simulink model "SmAHTR_r1_PITTRTNUKE"  (R2014a)
settings: Solver=ode4  StartTime=0.0  StopTime=250  FixedStep=.001  RelTol=1e-3
PreLoadFcn:
  | load DarkLowerCoeffs
  | load DarkMiddleCoeffs
  | load DarkUpperCoeffs
  | load breaks
values from neighbouring files (symbols this model uses):
  alpha = [ -2.61*pcm -0.53*pcm ]    [SmAHTR_Spatial_Kinetics.m]
  breaks = DarkLowerBreaks    [SmAHTR_Spatial_Kinetics.m]
  cpc = 2414    [SmAHTR_Spatial_Kinetics.m]
  cpp = 2414    [SmAHTR_Spatial_Kinetics.m]
  DarkLowerCoeffs = ppDarkLower.coefs    [SmAHTR_Spatial_Kinetics.m]
  DarkMiddleCoeffs = ppDarkMiddle.coefs    [SmAHTR_Spatial_Kinetics.m]
  DarkRodWorthInserted = -3*Beta    (= -0.00489)    [SmAHTR_Spatial_Kinetics.m]
  DarkUpperCoeffs = ppDarkUpper.coefs    [SmAHTR_Spatial_Kinetics.m]
  delta_t = 1 / sensor_sampling_rate    (= 0.001)    [HeatExchanger_ps.m]    (also in steady_data_76rssi_30_1.mat = 0.1; steady_data_76rssi_40.mat = 0.1; steady_data_76rssi_iter.mat = 0.1; steady_data_76rssi_iter_reduce.mat = 0.1)
  Kc1 = 1/(rho_secondary*V_secondary)    (= 0.00032726218348)    [SmAHTR_Spatial_Kinetics.m]
  Kc2 = (h_secondary*A)/(cps*rho_secondary*V_secondary)    (= 1.23242359038)    [SmAHTR_Spatial_Kinetics.m]
  Kh1 = 1/(rho_primary*V_primary)    (= 0.000447917898441)    [SmAHTR_Spatial_Kinetics.m]
  Kh2 = (h_primary*A)/(cpp*rho_primary*V_primary)    (= 1.29038206968)    [SmAHTR_Spatial_Kinetics.m]
  Kw1 = h_primary    (= 23800)    [SmAHTR_Spatial_Kinetics.m]
  Kw2 = h_secondary    (= 24500)    [SmAHTR_Spatial_Kinetics.m]
  Kw3 = A/(rho_tube*cpw*V_tube)    (= 0.000122049789882)    [SmAHTR_Spatial_Kinetics.m]
  L1 = .0124    (= 0.0124)    [SmAHTR_Spatial_Kinetics.m]
  L2 = .0305    (= 0.0305)    [SmAHTR_Spatial_Kinetics.m]
  rcp_activatetime = 20    [SmAHTR_Spatial_Kinetics.m]
  rcpt = 0.1    [SmAHTR_Spatial_Kinetics.m]
  SaltVaultICs = -AtempSALT\btempSALT*u0    [SmAHTR_Spatial_Kinetics.m]
  Tp_i = 700    [SmAHTR_Spatial_Kinetics.m]
  Ts_i = 600    [SmAHTR_Spatial_Kinetics.m]
  Tw_i = 650    [SmAHTR_Spatial_Kinetics.m]
  xfc0 = -Atemp\btemp*u0    [SmAHTR_Spatial_Kinetics.m]
libraries: powerlib_meascontrol x9, simulink x3
(part 1 of 2)
settings Model: BufferReuse=off  Creator=LabUser  LastModifiedBy=wangwenchen
settings DataIOCC: SignalLoggingSaveFormat=ModelDataLogs
settings OptimizationCC: BlockReduction=off  OptimizeBlockIOStorage=off  BufferReuse=off  GlobalBufferReuse=off  ExpressionFolding=off  LocalBlockOutputs=off
settings DebuggingCC: UnderspecifiedInitializationDetection=Classic  MultiTaskDSMMsg=warning  MultiTaskCondExecSysMsg=none  StateNameClashWarn=warning
settings HardwareCC: ProdIntDivRoundTo=Zero  ProdEndianess=LittleEndian  ProdHWDeviceType=Generic->32-bit x86 compatible
settings RTWCC: ProcessScript=grt_make_rtw_hook  IncludeERTFirstTime=on  RTWCompilerOptimization=On

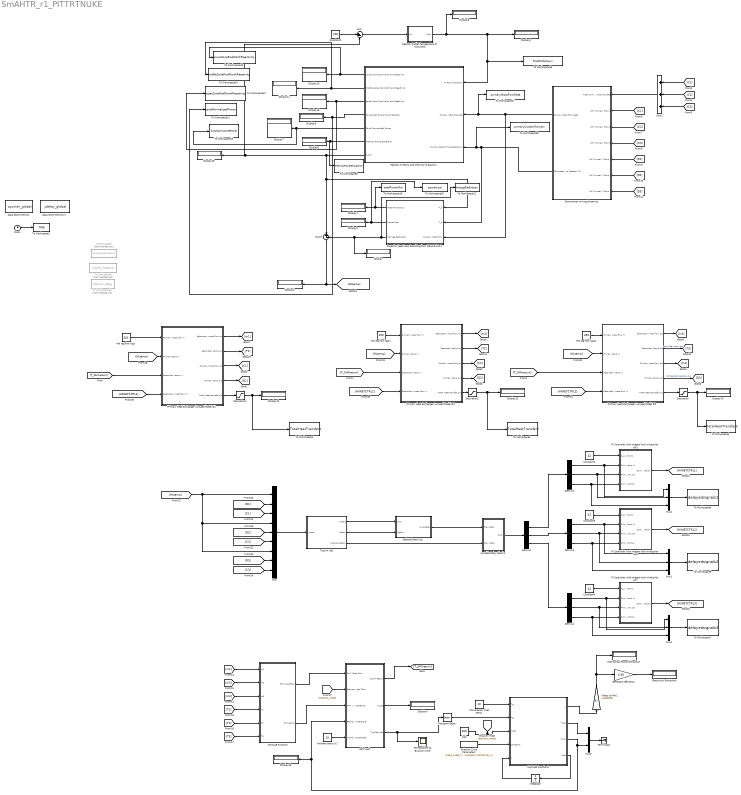
== system SmAHTR_r1_PITTRTNUKE ==
  Ambient temp (C) : Constant  Value=25
  Brayton Cycle Parameters : FromWorkspace  VariableName=[0,eta_C,eta_T,r,cpCO2Turbine,cpCO2Compressor,rhoCO2,tau_t]  SampleTime=0
  Clock : Clock
  Compressor Inlet Temp : Constant  Value=10
  Constant1 : Constant  Value=700
  Constant2 : Constant  Value=42
  Constant3 : Constant  Value=42
  Constant4 : Constant  Value=42
  Data Store Memory : DataStoreMemory  DataStoreName=counter_global  ReadBeforeWriteMsg=warning  WriteAfterWriteMsg=warning  WriteAfterReadMsg=warning  OutDataTypeStr=int32
  Data Store Memory1 : DataStoreMemory  DataStoreName=ydelay_global  ReadBeforeWriteMsg=warning  WriteAfterWriteMsg=warning  WriteAfterReadMsg=warning  InitialValue=ones(10,1)  OutDataTypeStr=int32
  Delayed Data Up2 : MATLAB Function  TreatAsAtomicUnit=on  SystemSampleTime=0.001
  Demux{1..4} (4 alike) : Demux  Outputs=3
  Display{,1..16,18} (18 alike) : Display
  Downcomer mixing dynamics : Subsystem
  Electricity Extraction : Display
  Generator Efficiency : Gain  Gain=0.60
  Hot leg flow kg/s : Constant  Value=350
  Hot leg flow kg/s1 : Constant  Value=350
  Hot leg flow kg/s2 : Constant  Value=350
  Integrator : Integrator
  MATLAB Function : MATLAB Function  TreatAsAtomicUnit=on
  MATLAB Function1 : MATLAB Function  TreatAsAtomicUnit=on
  Mechanical Power Extraction : Display
  Mux : Mux  Inputs=9
  Mux1 : Mux  Inputs=3
  Mux2 : Mux  Inputs=3
  Mux3 : Mux  Inputs=2
  Mux4 : Mux  Inputs=3
  PI Controller with Integral Anti-windup for HX5 : Subsystem
  PI Controller with Integral Anti-windup for HX6 : Subsystem
  PI Controller with Integral Anti-windup for HX7 : Subsystem
  Parasitic Heat Loss Resulting from DRACS HXs1 : Subsystem
  Primary Heat Exchanger Lumped Model #1 : Subsystem
  Primary Heat Exchanger Lumped Model #2 : Subsystem
  Primary Heat Exchanger Lumped Model #3 : Subsystem
  Reactor Kinetics and Thermal Hydraulics : Subsystem
  Reactor Outlet Temperature PI Controller : Subsystem
  Salt Vault : Subsystem
  Saturation : Saturate  UpperLimit=inf  LowerLimit=0
  Saturation1 : Saturate  UpperLimit=inf  LowerLimit=0
  Saturation2 : Saturate  UpperLimit=inf  LowerLimit=0
  Sum : Sum  Inputs=|+-
  Sum1 : Sum  Inputs=+++
  Sum3 : Sum  Inputs=|+-
  Temperature to Brayton cycle : Scope
      settings: SaveName=ScopeData5
  Terminator : Terminator
  To Workspace : ToWorkspace  Commented=on  VariableName=primarytempout  SaveFormat=Timeseries  SampleTime=-1
  To Workspace1 : ToWorkspace  VariableName=TIME  SampleTime=-1
  To Workspace10 : ToWorkspace  VariableName=ZonalNormalizedPower  SaveFormat=Timeseries  SampleTime=-1
  To Workspace11 : ToWorkspace  VariableName=zonalNormalizedPower  SaveFormat=Timeseries  SampleTime=-1
  To Workspace12 : ToWorkspace  VariableName=upperZoneRodWorthReactivity  SaveFormat=Timeseries  SampleTime=-1
  To Workspace13 : ToWorkspace  Commented=on  VariableName=network_delay  SampleTime=-1
  To Workspace14 : ToWorkspace  VariableName=middleZoneRodWorthReactivity  SaveFormat=Timeseries  SampleTime=-1
  To Workspace15 : ToWorkspace  VariableName=lowerZoneRodWorthReactivity  SaveFormat=Timeseries  SampleTime=-1
  To Workspace16 : ToWorkspace  VariableName=RodWithdrawn  SaveFormat=Timeseries  SampleTime=-1
  To Workspace17 : ToWorkspace  VariableName=primaryMassFlowRate  SaveFormat=Timeseries  SampleTime=-1
  To Workspace18 : ToWorkspace  VariableName=primaryCoolantTempIn  SaveFormat=Timeseries  SampleTime=-1
  To Workspace19 : ToWorkspace  VariableName=totalPowerOut  SaveFormat=Timeseries  SampleTime=-1
  To Workspace2 : ToWorkspace  VariableName=TotalHeatTransfer2  SaveFormat=Timeseries  SampleTime=-1
  To Workspace20 : ToWorkspace  VariableName=powerLost  SaveFormat=Timeseries  SampleTime=-1
  To Workspace21 : ToWorkspace  VariableName=hotLegReduction  SaveFormat=Timeseries  SampleTime=-1
  To Workspace3 : ToWorkspace  VariableName=TotalHeatTransfer1  SaveFormat=Timeseries  SampleTime=-1
  To Workspace4 : ToWorkspace  VariableName=TotalHeatTransfer3  SaveFormat=Timeseries  SampleTime=-1
  To Workspace5 : ToWorkspace  Commented=on  VariableName=Signal_measure  SampleTime=-1
  To Workspace6 : ToWorkspace  VariableName=delayedsignals1  SaveFormat=Timeseries  SampleTime=-1
  To Workspace7 : ToWorkspace  VariableName=delayedsignals3  SaveFormat=Timeseries  SampleTime=-1
  To Workspace8 : ToWorkspace  VariableName=delayedsignals2  SaveFormat=Timeseries  SampleTime=-1
  To Workspace9 : ToWorkspace  VariableName=ThermalPowerExtraction  SaveFormat=Timeseries  SampleTime=-1
  Tossim Up1 : MATLAB Function  TreatAsAtomicUnit=on  SystemSampleTime=0.001
  Transport Delay : TransportDelay  DelayTime=0.5  BufferSize=3072
  Variable Delay Block1 : Subsystem
  Watts to MW1 : Gain  Gain=1/1000000
  kg/s : Constant  Value=300
  wires:
  Reactor Outlet Temperature PI Controller/1(Out1) -> Reactor Kinetics and Thermal Hydraulics/1(% Rod Withdrawn), To Workspace16/1, Display5/1, Display8/1
  Downcomer mixing dynamics/1(Primary Mass Flow Rate) -> Parasitic Heat Loss Resulting from DRACS HXs1/3(Primary Mass Flow), To Workspace17/1, Reactor Kinetics and Thermal Hydraulics/2(Primary Mass Flowrate)
  Parasitic Heat Loss Resulting from DRACS HXs1/3(Hot Leg Reduction) -> Sum3/2, Display/1, To Workspace21/1
  Parasitic Heat Loss Resulting from DRACS HXs1/1(Total Power Out) -> To Workspace19/1, Display1/1
  Parasitic Heat Loss Resulting from DRACS HXs1/2(Power Lost) -> To Workspace20/1, Display2/1
  Reactor Kinetics and Thermal Hydraulics/7(T_hot) -> Display16/1, Sum/2, Sum3/1, Parasitic Heat Loss Resulting from DRACS HXs1/1(T_h)
  Sum3/1 -> Display3/1, [HLtemp]
  Sum1/1 -> Downcomer mixing dynamics/1(Total primary mass flowrate)
  [C1] -> Sum1/1
  [C2] -> Sum1/2
  [C3] -> Sum1/3
  [C1] -> Downcomer mixing dynamics/2(PHX Primary Flow 1)
  [C2] -> Downcomer mixing dynamics/3(PHX Primary Flow 2)
  [C3] -> Downcomer mixing dynamics/4(PHX Primary Flow 3)
  [D1] -> Downcomer mixing dynamics/5(PHX Primary Temp 1)
  [D2] -> Downcomer mixing dynamics/6(PHX Primary Temp 2)
  [D3] -> Downcomer mixing dynamics/7(PHX Primary Temp 3)
  Downcomer mixing dynamics/2(Temperature to Reactor T-H) -> Parasitic Heat Loss Resulting from DRACS HXs1/2(T_c), To Workspace18/1, Reactor Kinetics and Thermal Hydraulics/3(Primary Coolant Temperature In)
  Hot leg flow kg/s/1 -> Primary Heat Exchanger Lumped Model #1/1(Primary mass flow in)
  Primary Heat Exchanger Lumped Model #1/3(Primary mass flow out) -> [C1]
  Primary Heat Exchanger Lumped Model #1/1(Secondary mass flow out) -> [m1]
  Primary Heat Exchanger Lumped Model #1/2(Secondary temp out) -> [T1]
  Hot leg flow kg/s1/1 -> Primary Heat Exchanger Lumped Model #2/1(Primary mass flow in)
  Primary Heat Exchanger Lumped Model #2/3(Primary mass flow out) -> [C2]
  Primary Heat Exchanger Lumped Model #1/4(Primary temp out) -> [D1]
  Primary Heat Exchanger Lumped Model #2/4(Primary temp out) -> [D2]
  Primary Heat Exchanger Lumped Model #2/1(Secondary mass flow out) -> [m2]
  Primary Heat Exchanger Lumped Model #2/2(Secondary temp out) -> [T2]
  Primary Heat Exchanger Lumped Model #3/2(Secondary temp out) -> [T3]  "cold leg  temp out"
  Primary Heat Exchanger Lumped Model #3/4(Primary temp out) -> [D3]  "hot leg temperature out"
  Hot leg flow kg/s2/1 -> Primary Heat Exchanger Lumped Model #3/1(Primary mass flow in)
  Primary Heat Exchanger Lumped Model #3/1(Secondary mass flow out) -> [m3]
  Primary Heat Exchanger Lumped Model #3/3(Primary mass flow out) -> [C3]
  Primary Heat Exchanger Lumped Model #2/5("Total Heat transfer out ") -> Saturation2/1
  [HLtemp] -> Primary Heat Exchanger Lumped Model #1/2(Primary temp in)
  [HLtemp] -> Primary Heat Exchanger Lumped Model #2/2(Primary temp in)
  [HLtemp] -> Primary Heat Exchanger Lumped Model #3/2(Primary temp in)
  Primary Heat Exchanger Lumped Model #1/5("Total Heat transfer out ") -> Saturation1/1
  Primary Heat Exchanger Lumped Model #3/5("Total Heat transfer out ") -> Saturation/1
  Saturation/1 -> To Workspace4/1, Display14/1
  Saturation1/1 -> To Workspace3/1, Display12/1
  Saturation2/1 -> To Workspace2/1, Display13/1
  Salt Vault/1(T_SHX Return) -> [T_SHXreturn]
  Salt Vault/3(T_to Brayton) -> Transport Delay/1, Temperature to Brayton cycle/1
  [m1] -> MATLAB Function/1(m1)
  [m2] -> MATLAB Function/2(m2)
  [m3] -> MATLAB Function/3(m3)
  [T1] -> MATLAB Function/4(T1)
  [T2] -> MATLAB Function/5(T2)
  [T3] -> MATLAB Function/6(T3)
  MATLAB Function/1(SHX_massflow) -> Salt Vault/1(SHX Mass Flow)
  [brayton_mdot] -> Salt Vault/2(Brayton Mass Flow)
  MATLAB Function/2(SHX_temp) -> Salt Vault/3(SHX Inlet Temperature)
  Salt Vault/2(T_salt) -> Display4/1
  MATLAB Function1/4(xdot) -> Integrator/1
  Integrator/1 -> MATLAB Function1/5(x)
  kg/s/1 -> [brayton_mdot], MATLAB Function1/3(mdot)
  Compressor Inlet Temp/1 -> MATLAB Function1/1(Tc_i)
  MATLAB Function1/1(y) -> Watts to MW1/1
  MATLAB Function1/2(Tt_o) -> Mux3/1
  MATLAB Function1/3(Tc_o) -> Display18/1, Salt Vault/4(Brayton Inlet Temperature), Mux3/2
  Transport Delay/1 -> MATLAB Function1/2(Tt_i)
  Watts to MW1/1 -> Generator Efficiency/1, Mechanical Power Extraction/1
  Generator Efficiency/1 -> Electricity Extraction/1
  Ambient temp (C)/1 -> Salt Vault/5(Ambient Temperatre)
  Brayton Cycle Parameters/1 -> MATLAB Function1/4(constants)
  Reactor Kinetics and Thermal Hydraulics/6(Thermal Power Extraction) -> To Workspace9/1, Display6/1
  Reactor Kinetics and Thermal Hydraulics/5(Zonal Normalized Power) -> To Workspace10/1, Display7/1
  Reactor Kinetics and Thermal Hydraulics/1(Lower Zone Rod Worth and Reactivity) -> To Workspace15/1, Display10/1
  Reactor Kinetics and Thermal Hydraulics/2(Middle Zone Rod Worth and Reactivity) -> To Workspace14/1, Display11/1
  Reactor Kinetics and Thermal Hydraulics/3(Upper Zone Rod Worth and Reactivity) -> To Workspace12/1, Display15/1
  Mux3/1 -> Terminator/1
  [T_SHXreturn] -> Primary Heat Exchanger Lumped Model #1/3(Secondary temp in)
  [T_SHXreturn] -> Primary Heat Exchanger Lumped Model #2/3(Secondary temp in)
  [T_SHXreturn] -> Primary Heat Exchanger Lumped Model #3/3(Secondary temp in)
  Sum/1 -> Reactor Outlet Temperature PI Controller/1(In1)
  Constant1/1 -> Sum/1
  Clock/1 -> To Workspace1/1
  [HLtemp] -> Mux/1, Mux/4, Mux/7
  [C1] -> Mux/3
  [C2] -> Mux/6
  [C3] -> Mux/9
  [D1] -> Mux/2
  [D2] -> Mux/5
  [D3] -> Mux/8
  Mux/1 -> Tossim Up1/1(ymea)
  Tossim Up1/1(ymea1) -> Delayed Data Up2/1(yout)
  Tossim Up1/2(ydelay) -> Delayed Data Up2/2(ydelay)
  Tossim Up1/3(ynetwork_delay) -> Variable Delay Block1/2(Delay vector)
  Delayed Data Up2/1(yout_delay) -> Variable Delay Block1/1(Signal vector)
  Constant2/1 -> PI Controller with Integral Anti-windup for HX5/1(P_demand (MW)2)
  Constant3/1 -> PI Controller with Integral Anti-windup for HX6/1(P_demand (MW)2)
  Constant4/1 -> PI Controller with Integral Anti-windup for HX7/1(P_demand (MW)2)
  Variable Delay Block1/1(Out1) -> Demux1/1
  Demux1/1 -> Demux2/1
  Demux1/2 -> Demux3/1
  Demux1/3 -> Demux4/1
  Demux2/3 -> Mux2/3, PI Controller with Integral Anti-windup for HX5/4(Primary mass flow)
  Demux2/1 -> Mux2/1, PI Controller with Integral Anti-windup for HX5/2(Primary temp in)
  Demux2/2 -> Mux2/2, PI Controller with Integral Anti-windup for HX5/3(Primary temp out)
  Demux3/1 -> Mux1/1, PI Controller with Integral Anti-windup for HX6/2(Primary temp in)
  Demux3/2 -> Mux1/2, PI Controller with Integral Anti-windup for HX6/3(Primary temp out)
  Demux3/3 -> Mux1/3, PI Controller with Integral Anti-windup for HX6/4(Primary mass flow)
  Demux4/2 -> Mux4/2, PI Controller with Integral Anti-windup for HX7/3(Primary temp out)
  Demux4/3 -> Mux4/3, PI Controller with Integral Anti-windup for HX7/4(Primary mass flow)
  [HXNETCTRL1] -> Primary Heat Exchanger Lumped Model #1/4(Secondary mass flow in)
  [HXNETCTRL2] -> Primary Heat Exchanger Lumped Model #2/4(Secondary mass flow in)
  [HXNETCTRL3] -> Primary Heat Exchanger Lumped Model #3/4(Secondary mass flow in)
  PI Controller with Integral Anti-windup for HX5/1(Control Action) -> [HXNETCTRL1]
  PI Controller with Integral Anti-windup for HX6/1(Control Action) -> [HXNETCTRL2]
  PI Controller with Integral Anti-windup for HX7/1(Control Action) -> [HXNETCTRL3]
  Mux1/1 -> To Workspace8/1
  Mux2/1 -> To Workspace6/1
  Demux4/1 -> Mux4/1, PI Controller with Integral Anti-windup for HX7/2(Primary temp in)
  Mux4/1 -> To Workspace7/1
  Reactor Kinetics and Thermal Hydraulics/4(Normalized Power Out of Reactor) -> To Workspace11/1, Display9/1

== system SmAHTR_r1_PITTRTNUKE/Downcomer mixing dynamics ==
  Total primary mass flowrate : Inport
  PHX Primary Flow 1 : Inport  Port=2
  PHX Primary Flow 2 : Inport  Port=3
  PHX Primary Flow 3 : Inport  Port=4
  PHX Primary Temp 1 : Inport  Port=5
  PHX Primary Temp 2 : Inport  Port=6
  PHX Primary Temp 3 : Inport  Port=7
  MATLAB Function : MATLAB Function  TreatAsAtomicUnit=on
  Primary Mass Flow Rate : Outport
  Temperature to Reactor T-H : Outport  Port=2
  wires:
  Total primary mass flowrate/1 -> MATLAB Function/1(a)
  PHX Primary Flow 1/1 -> MATLAB Function/2(b)
  PHX Primary Flow 2/1 -> MATLAB Function/3(c)
  PHX Primary Flow 3/1 -> MATLAB Function/4(d)
  PHX Primary Temp 1/1 -> MATLAB Function/5(e)
  PHX Primary Temp 2/1 -> MATLAB Function/6(f)
  PHX Primary Temp 3/1 -> MATLAB Function/7(g)
  MATLAB Function/1(y) -> Temperature to Reactor T-H/1
  MATLAB Function/2(z) -> Primary Mass Flow Rate/1

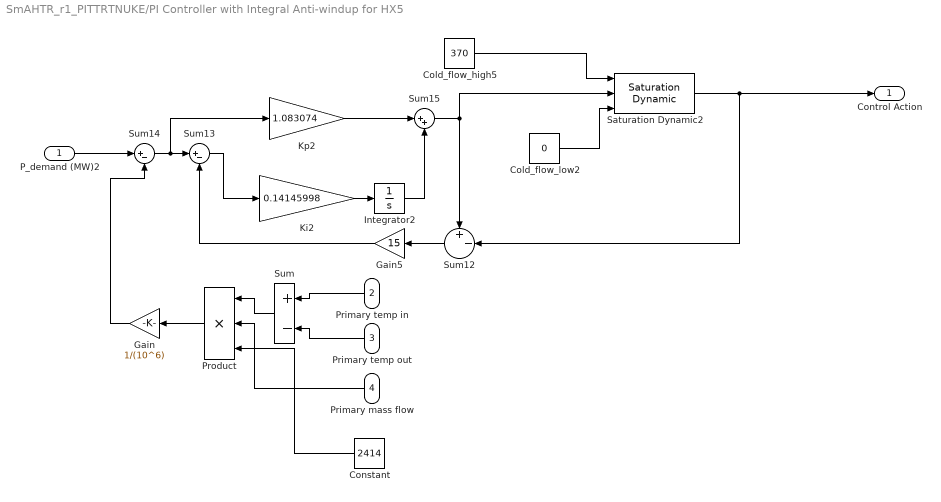
== system SmAHTR_r1_PITTRTNUKE/PI Controller with Integral Anti-windup for HX5 ==
  P_demand (MW)2 : Inport
  Primary temp in : Inport  Port=2
  Primary temp out : Inport  Port=3
  Primary mass flow : Inport  Port=4
  Cold_flow_high5 : Constant  Value=370
  Cold_flow_low2 : Constant  Value=0
  Constant : Constant  Value=2414
  Gain : Gain  Gain=1/(10^6)
  Gain5 : Gain  Gain=15
  Integrator2 : Integrator  InitialCondition=100
  Ki2 : Gain  Gain=0.14145998
  Kp2 : Gain  Gain=1.083074
  Product : Product  Inputs=3
  Saturation Dynamic2 : simulink/Discontinuities/Saturation Dynamic  OutMin=[]  OutMax=[]  OutDataTypeStr=Inherit: Same as second input  OutDataType=fixdt(1, 16)  OutScaling=2^-10  DoSatur=off
  Sum : Sum  Inputs=+-
  Sum12 : Sum  Inputs=+-|
  Sum13 : Sum  Inputs=|+-
  Sum14 : Sum  Inputs=|+-
  Sum15 : Sum  Inputs=|++
  Control Action : Outport
  wires:
  Product/1 -> Gain/1
  Cold_flow_low2/1 -> Saturation Dynamic2/3
  Cold_flow_high5/1 -> Saturation Dynamic2/1
  Sum14/1 -> Kp2/1, Sum13/1
  P_demand (MW)2/1 -> Sum14/1
  Sum12/1 -> Gain5/1
  Integrator2/1 -> Sum15/2
  Gain5/1 -> Sum13/2
  Sum13/1 -> Ki2/1
  Ki2/1 -> Integrator2/1
  Kp2/1 -> Sum15/1
  Saturation Dynamic2/1 -> Control Action/1, Sum12/2
  Sum15/1 -> Sum12/1, Saturation Dynamic2/2
  Primary temp in/1 -> Sum/1
  Primary temp out/1 -> Sum/2
  Sum/1 -> Product/1
  Primary mass flow/1 -> Product/2
  Constant/1 -> Product/3
  Gain/1 -> Sum14/2

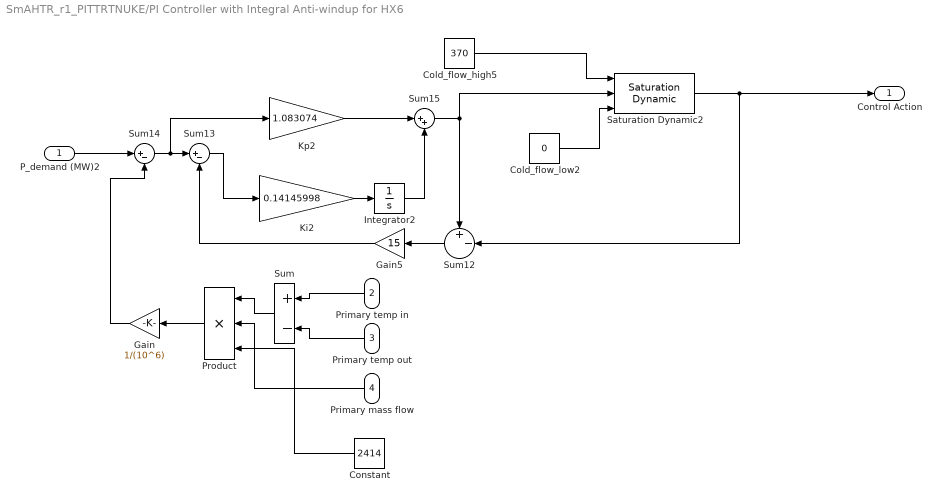
== system SmAHTR_r1_PITTRTNUKE/PI Controller with Integral Anti-windup for HX6 ==
  P_demand (MW)2 : Inport
  Primary temp in : Inport  Port=2
  Primary temp out : Inport  Port=3
  Primary mass flow : Inport  Port=4
  Cold_flow_high5 : Constant  Value=370
  Cold_flow_low2 : Constant  Value=0
  Constant : Constant  Value=2414
  Gain : Gain  Gain=1/(10^6)
  Gain5 : Gain  Gain=15
  Integrator2 : Integrator  InitialCondition=100
  Ki2 : Gain  Gain=0.14145998
  Kp2 : Gain  Gain=1.083074
  Product : Product  Inputs=3
  Saturation Dynamic2 : simulink/Discontinuities/Saturation Dynamic  OutMin=[]  OutMax=[]  OutDataTypeStr=Inherit: Same as second input  OutDataType=fixdt(1, 16)  OutScaling=2^-10  DoSatur=off
  Sum : Sum  Inputs=+-
  Sum12 : Sum  Inputs=+-|
  Sum13 : Sum  Inputs=|+-
  Sum14 : Sum  Inputs=|+-
  Sum15 : Sum  Inputs=|++
  Control Action : Outport
  wires:
  Product/1 -> Gain/1
  Cold_flow_low2/1 -> Saturation Dynamic2/3
  Cold_flow_high5/1 -> Saturation Dynamic2/1
  Sum14/1 -> Kp2/1, Sum13/1
  P_demand (MW)2/1 -> Sum14/1
  Sum12/1 -> Gain5/1
  Integrator2/1 -> Sum15/2
  Gain5/1 -> Sum13/2
  Sum13/1 -> Ki2/1
  Ki2/1 -> Integrator2/1
  Kp2/1 -> Sum15/1
  Saturation Dynamic2/1 -> Control Action/1, Sum12/2
  Sum15/1 -> Sum12/1, Saturation Dynamic2/2
  Primary temp in/1 -> Sum/1
  Primary temp out/1 -> Sum/2
  Sum/1 -> Product/1
  Primary mass flow/1 -> Product/2
  Constant/1 -> Product/3
  Gain/1 -> Sum14/2

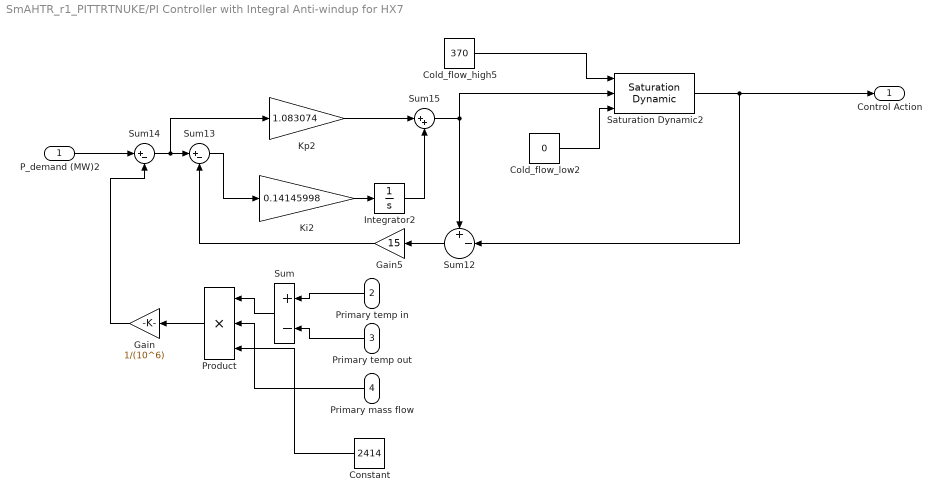
== system SmAHTR_r1_PITTRTNUKE/PI Controller with Integral Anti-windup for HX7 ==
  P_demand (MW)2 : Inport
  Primary temp in : Inport  Port=2
  Primary temp out : Inport  Port=3
  Primary mass flow : Inport  Port=4
  Cold_flow_high5 : Constant  Value=370
  Cold_flow_low2 : Constant  Value=0
  Constant : Constant  Value=2414
  Gain : Gain  Gain=1/(10^6)
  Gain5 : Gain  Gain=15
  Integrator2 : Integrator  InitialCondition=100
  Ki2 : Gain  Gain=0.14145998
  Kp2 : Gain  Gain=1.083074
  Product : Product  Inputs=3
  Saturation Dynamic2 : simulink/Discontinuities/Saturation Dynamic  OutMin=[]  OutMax=[]  OutDataTypeStr=Inherit: Same as second input  OutDataType=fixdt(1, 16)  OutScaling=2^-10  DoSatur=off
  Sum : Sum  Inputs=+-
  Sum12 : Sum  Inputs=+-|
  Sum13 : Sum  Inputs=|+-
  Sum14 : Sum  Inputs=|+-
  Sum15 : Sum  Inputs=|++
  Control Action : Outport
  wires:
  Product/1 -> Gain/1
  Cold_flow_low2/1 -> Saturation Dynamic2/3
  Cold_flow_high5/1 -> Saturation Dynamic2/1
  Sum14/1 -> Kp2/1, Sum13/1
  P_demand (MW)2/1 -> Sum14/1
  Sum12/1 -> Gain5/1
  Integrator2/1 -> Sum15/2
  Gain5/1 -> Sum13/2
  Sum13/1 -> Ki2/1
  Ki2/1 -> Integrator2/1
  Kp2/1 -> Sum15/1
  Saturation Dynamic2/1 -> Control Action/1, Sum12/2
  Sum15/1 -> Sum12/1, Saturation Dynamic2/2
  Primary temp in/1 -> Sum/1
  Primary temp out/1 -> Sum/2
  Sum/1 -> Product/1
  Primary mass flow/1 -> Product/2
  Constant/1 -> Product/3
  Gain/1 -> Sum14/2

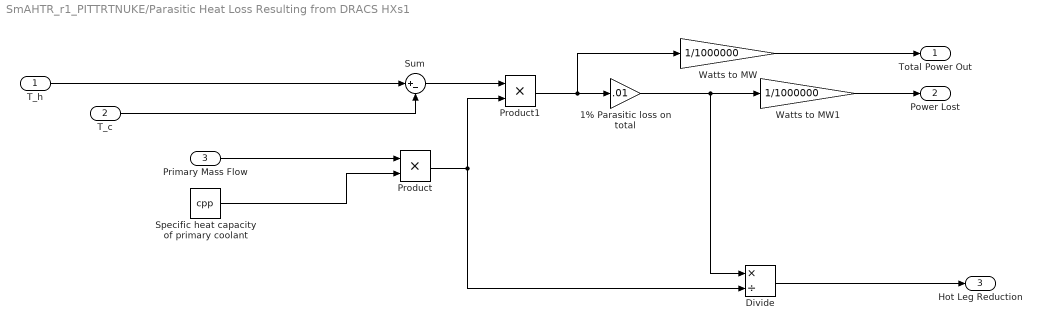
== system SmAHTR_r1_PITTRTNUKE/Parasitic Heat Loss Resulting from DRACS HXs1 ==
  T_h : Inport
  T_c : Inport  Port=2
  Primary Mass Flow : Inport  Port=3
  1% Parasitic loss on total : Gain  Gain=.01
  Divide : Product  Inputs=*/
  Product : Product
  Product1 : Product
  Specific heat capacity of primary coolant : Constant  Value=cpp
  Sum : Sum  Inputs=|+-
  Watts to MW : Gain  Gain=1/1000000
  Watts to MW1 : Gain  Gain=1/1000000
  Total Power Out : Outport
  Power Lost : Outport  Port=2
  Hot Leg Reduction : Outport  Port=3
  wires:
  Primary Mass Flow/1 -> Product/1
  Specific heat capacity of primary coolant/1 -> Product/2
  T_c/1 -> Sum/2
  Sum/1 -> Product1/1
  Product/1 -> Product1/2, Divide/2
  Product1/1 -> Watts to MW/1, 1% Parasitic loss on total/1
  Watts to MW/1 -> Total Power Out/1
  1% Parasitic loss on total/1 -> Divide/1, Watts to MW1/1
  Watts to MW1/1 -> Power Lost/1
  T_h/1 -> Sum/1
  Divide/1 -> Hot Leg Reduction/1

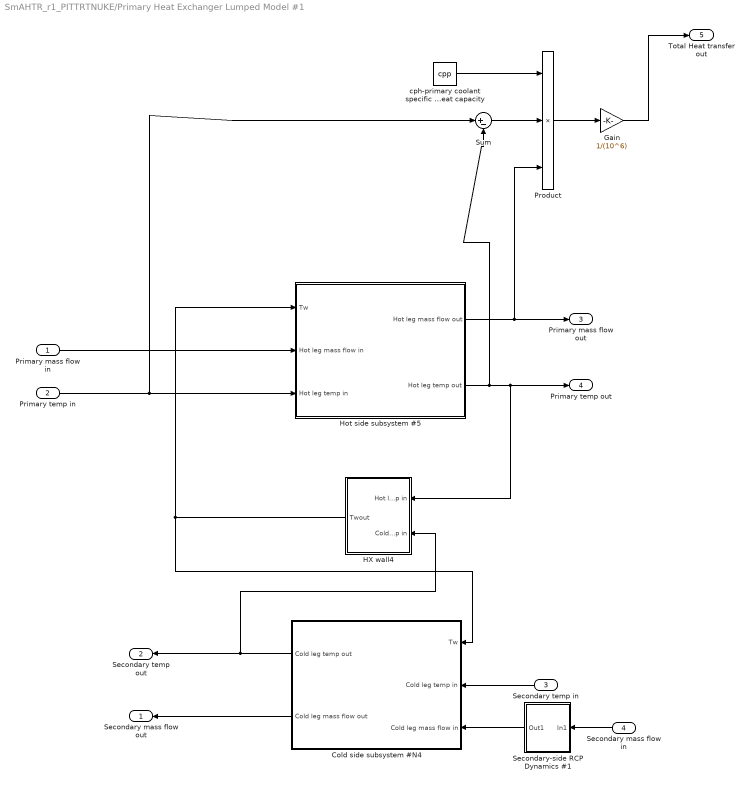
== system SmAHTR_r1_PITTRTNUKE/Primary Heat Exchanger Lumped Model #1 ==
  Primary mass flow in : Inport
  Primary temp in : Inport  Port=2
  Secondary temp in : Inport  Port=3
  Secondary mass flow in : Inport  Port=4
  Cold side subsystem #N4 : Subsystem
  Gain : Gain  Gain=1/(10^6)
  HX wall4 : Subsystem
  Hot side subsystem #5 : Subsystem
  Product : Product  Inputs=3
  Secondary-side RCP Dynamics #1 : Subsystem
  Sum : Sum  Inputs=|+-
  cph-primary coolant specific heat capacity : Constant  Value=cpp
  Secondary mass flow out : Outport
  Secondary temp out : Outport  Port=2
  Primary mass flow out : Outport  Port=3
  Primary temp out : Outport  Port=4
  "Total Heat transfer out " : Outport  Port=5
  wires:
  Cold side subsystem #N4/1(Cold leg temp out) -> Secondary temp out/1, HX wall4/2(Cold leg temp in)
  Cold side subsystem #N4/2(Cold leg mass flow out) -> Secondary mass flow out/1
  Primary mass flow in/1 -> Hot side subsystem #5/2(Hot leg mass flow in)
  Primary temp in/1 -> Hot side subsystem #5/3(Hot leg temp in), Sum/1
  Secondary mass flow in/1 -> Secondary-side RCP Dynamics #1/1(In1)
  Secondary temp in/1 -> Cold side subsystem #N4/2(Cold leg temp in)
  HX wall4/1(Twout) -> Cold side subsystem #N4/1(Tw), Hot side subsystem #5/1(Tw)
  Hot side subsystem #5/1(Hot leg mass flow out) -> Product/3, Primary mass flow out/1
  Hot side subsystem #5/2(Hot leg temp out) -> HX wall4/1(Hot leg temp in), Primary temp out/1, Sum/2
  cph-primary coolant specific heat capacity/1 -> Product/1
  Sum/1 -> Product/2
  Product/1 -> Gain/1
  Gain/1 -> "Total Heat transfer out "/1
  Secondary-side RCP Dynamics #1/1(Out1) -> Cold side subsystem #N4/3(Cold leg mass flow in)

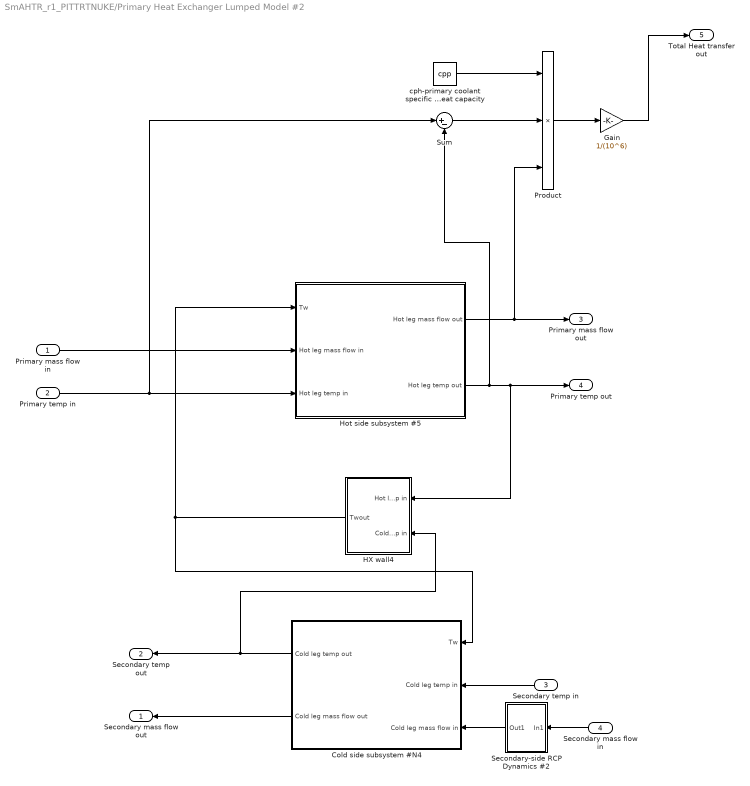
== system SmAHTR_r1_PITTRTNUKE/Primary Heat Exchanger Lumped Model #2 ==
  Primary mass flow in : Inport
  Primary temp in : Inport  Port=2
  Secondary temp in : Inport  Port=3
  Secondary mass flow in : Inport  Port=4
  Cold side subsystem #N4 : Subsystem
  Gain : Gain  Gain=1/(10^6)
  HX wall4 : Subsystem
  Hot side subsystem #5 : Subsystem
  Product : Product  Inputs=3
  Secondary-side RCP Dynamics #2 : Subsystem
  Sum : Sum  Inputs=|+-
  cph-primary coolant specific heat capacity : Constant  Value=cpp
  Secondary mass flow out : Outport
  Secondary temp out : Outport  Port=2
  Primary mass flow out : Outport  Port=3
  Primary temp out : Outport  Port=4
  "Total Heat transfer out " : Outport  Port=5
  wires:
  Cold side subsystem #N4/1(Cold leg temp out) -> Secondary temp out/1, HX wall4/2(Cold leg temp in)
  Cold side subsystem #N4/2(Cold leg mass flow out) -> Secondary mass flow out/1
  Primary mass flow in/1 -> Hot side subsystem #5/2(Hot leg mass flow in)
  Primary temp in/1 -> Hot side subsystem #5/3(Hot leg temp in), Sum/1
  Secondary mass flow in/1 -> Secondary-side RCP Dynamics #2/1(In1)
  Secondary temp in/1 -> Cold side subsystem #N4/2(Cold leg temp in)
  HX wall4/1(Twout) -> Cold side subsystem #N4/1(Tw), Hot side subsystem #5/1(Tw)
  Hot side subsystem #5/1(Hot leg mass flow out) -> Product/3, Primary mass flow out/1
  Hot side subsystem #5/2(Hot leg temp out) -> HX wall4/1(Hot leg temp in), Primary temp out/1, Sum/2
  cph-primary coolant specific heat capacity/1 -> Product/1
  Sum/1 -> Product/2
  Product/1 -> Gain/1
  Gain/1 -> "Total Heat transfer out "/1
  Secondary-side RCP Dynamics #2/1(Out1) -> Cold side subsystem #N4/3(Cold leg mass flow in)

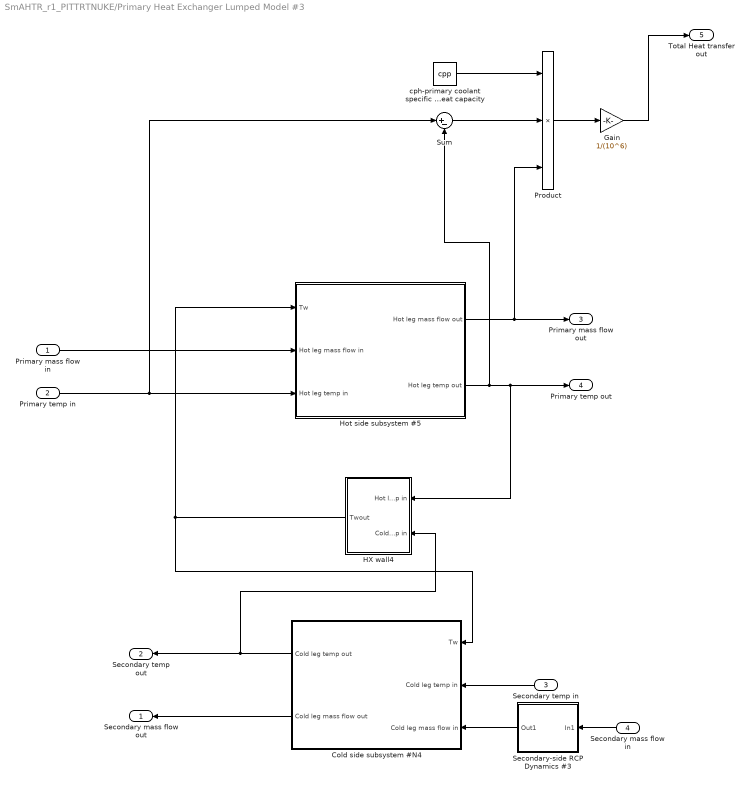
== system SmAHTR_r1_PITTRTNUKE/Primary Heat Exchanger Lumped Model #3 ==
  Primary mass flow in : Inport
  Primary temp in : Inport  Port=2
  Secondary temp in : Inport  Port=3
  Secondary mass flow in : Inport  Port=4
  Cold side subsystem #N4 : Subsystem
  Gain : Gain  Gain=1/(10^6)
  HX wall4 : Subsystem
  Hot side subsystem #5 : Subsystem
  Product : Product  Inputs=3
  Secondary-side RCP Dynamics #3 : Subsystem
  Sum : Sum  Inputs=|+-
  cph-primary coolant specific heat capacity : Constant  Value=cpp
  Secondary mass flow out : Outport
  Secondary temp out : Outport  Port=2
  Primary mass flow out : Outport  Port=3
  Primary temp out : Outport  Port=4
  "Total Heat transfer out " : Outport  Port=5
  wires:
  Cold side subsystem #N4/1(Cold leg temp out) -> Secondary temp out/1, HX wall4/2(Cold leg temp in)
  Cold side subsystem #N4/2(Cold leg mass flow out) -> Secondary mass flow out/1
  Primary mass flow in/1 -> Hot side subsystem #5/2(Hot leg mass flow in)
  Primary temp in/1 -> Hot side subsystem #5/3(Hot leg temp in), Sum/1
  Secondary mass flow in/1 -> Secondary-side RCP Dynamics #3/1(In1)
  Secondary temp in/1 -> Cold side subsystem #N4/2(Cold leg temp in)
  HX wall4/1(Twout) -> Cold side subsystem #N4/1(Tw), Hot side subsystem #5/1(Tw)
  Hot side subsystem #5/1(Hot leg mass flow out) -> Product/3, Primary mass flow out/1
  Hot side subsystem #5/2(Hot leg temp out) -> HX wall4/1(Hot leg temp in), Primary temp out/1, Sum/2
  cph-primary coolant specific heat capacity/1 -> Product/1
  Sum/1 -> Product/2
  Product/1 -> Gain/1
  Gain/1 -> "Total Heat transfer out "/1
  Secondary-side RCP Dynamics #3/1(Out1) -> Cold side subsystem #N4/3(Cold leg mass flow in)

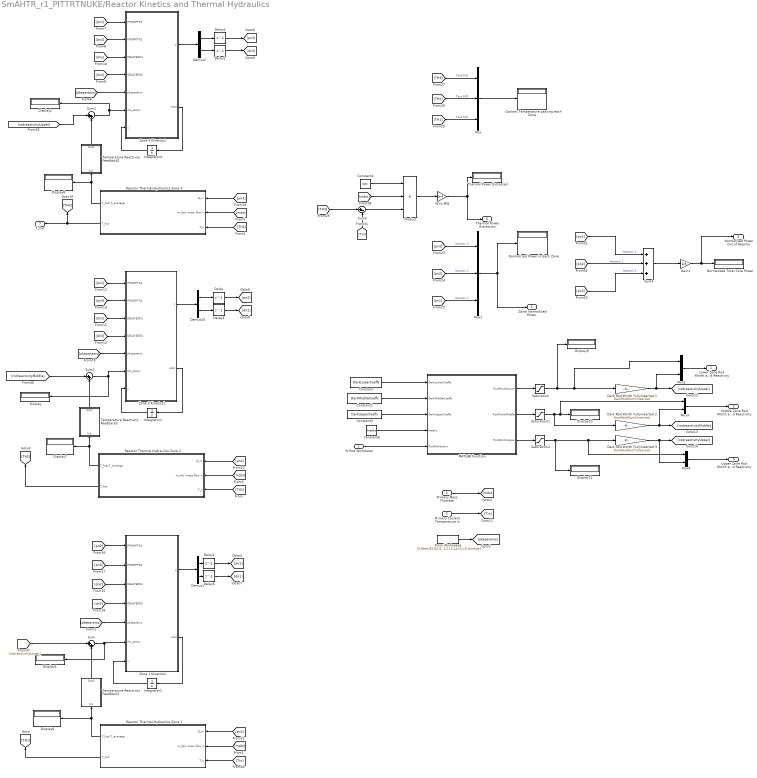
== system SmAHTR_r1_PITTRTNUKE/Reactor Kinetics and Thermal Hydraulics ==
  % Rod Withdrawn : Inport
  Primary Mass Flowrate : Inport  Port=2
  Primary Coolant Temperature In : Inport  Port=3
  Constant : Constant  Value=DarkLowerCoeffs
  Constant1 : Constant  Value=DarkMiddleCoeffs
  Constant3 : Constant  Value=DarkUpperCoeffs
  Constant4 : Constant  Value=cpc
  Constant6 : Constant  Value=breaks
  Coolant Temperature Leaving each Zone : Display
  Dark Rod Worth FullyInserted 1 : Gain  Gain=DarkRodWorthInserted
  Dark Rod Worth FullyInserted 2 : Gain  Gain=DarkRodWorthInserted
  Dark Rod Worth FullyInserted 3 : Gain  Gain=DarkRodWorthInserted
  Delay{,1..5} (6 alike) : Delay  DelayLength=1  InitialCondition=0
  Demux1 : Demux  Outputs=2
  Demux10 : Demux  Outputs=2
  Demux2 : Demux  Outputs=2
  Display{,1,4,6..11} (9 alike) : Display
  From Workspace : FromWorkspace  VariableName=[0,Beta,B1,B2,B3,B4,B5,B6,L1,L2,L3,L4,L5,L6,lambda]  SampleTime=0
  Gain1 : Gain  Gain=1/3
  Integrator1 : Integrator  InitialCondition=[1,L1,L2]
  Integrator2 : Integrator  InitialCondition=[1,L1,L2]
  Integrator4 : Integrator  InitialCondition=[1,L1,L2]
  MATLAB Function : MATLAB Function  TreatAsAtomicUnit=on
  Mux : Mux  Inputs=3
  Mux1 : Mux  Inputs=3
  Mux2 : Mux  Inputs=2
  Mux3 : Mux  Inputs=2
  Mux4 : Mux  Inputs=2
  Normalized Power in Each Zone : Display
  Normalized Total Core Power : Display
  Product : Product  Inputs=3
  Reactor Thermal-Hydraulics Zone 1 : Subsystem
  Reactor Thermal-Hydraulics Zone 2 : Subsystem
  Reactor Thermal-Hydraulics Zone 3 : Subsystem
  Saturation : Saturate  UpperLimit=inf  LowerLimit=0
  Saturation1 : Saturate  UpperLimit=inf  LowerLimit=0
  Saturation2 : Saturate  UpperLimit=inf  LowerLimit=0
  Sum : Sum  Inputs=|++
  Sum1 : Sum  Inputs=|++
  Sum2 : Sum  Inputs=|++
  Sum3 : Sum  Inputs=|+-
  Sum4 : Sum  Inputs=+++
  Temperature Reactivity Feedback1 : Subsystem
  Temperature Reactivity Feedback2 : Subsystem
  Temperature Reactivity Feedback3 : Subsystem
  Thermal Power Extracted : Display
  W to MW : Gain  Gain=1e-6
  Zone 1 Kinetics1 : MATLAB Function  TreatAsAtomicUnit=on
  Zone 2 Kinetics1 : MATLAB Function  TreatAsAtomicUnit=on
  Zone 3 Kinetics1 : MATLAB Function  TreatAsAtomicUnit=on
  Lower Zone Rod Worth and Reactivity : Outport
  Middle Zone Rod Worth and Reactivity : Outport  Port=2
  Upper Zone Rod Worth and Reactivity : Outport  Port=3
  Normalized Power Out of Reactor : Outport  Port=4
  Zonal Normalized Power : Outport  Port=5
  Thermal Power Extraction : Outport  Port=6
  T_hot : Outport  Port=7
  wires:
  [pkeparams] -> Zone 2 Kinetics1/5(pkeparams)
  Demux1/2 -> Delay5/1
  From Workspace/1 -> [pkeparams]
  Reactor Thermal-Hydraulics Zone 2/1(T_fuel,T_average) -> Display7/1, Temperature Reactivity Feedback3/1(In1)
  [TH1] -> Reactor Thermal-Hydraulics Zone 2/3(T_c)
  Temperature Reactivity Feedback3/1(Out1) -> Sum1/2
  [pkeparams] -> Zone 1 Kinetics1/5(pkeparams)
  Zone 1 Kinetics1/1(y) -> Demux1/1
  Reactor Thermal-Hydraulics Zone 1/1(T_fuel,T_average) -> Temperature Reactivity Feedback1/1(In1), Display6/1
  Temperature Reactivity Feedback1/1(Out1) -> Sum/2
  Demux1/1 -> Delay1/1
  Sum/1 -> Zone 1 Kinetics1/6(rho_temp), Display4/1
  [rodreactivityLower] -> Sum/1
  Sum1/1 -> Zone 2 Kinetics1/6(rho_temp), Display/1
  [rodreactivityMiddle] -> Sum1/1
  Mux/1 -> Coolant Temperature Leaving each Zone/1
  Reactor Thermal-Hydraulics Zone 1/2(T_hot) -> [TH1]
  [mdot] -> Reactor Thermal-Hydraulics Zone 2/2(m_dot -mass flow in)
  [mdot] -> Reactor Thermal-Hydraulics Zone 1/2(m_dot -mass flow in)
  Reactor Thermal-Hydraulics Zone 3/1(T_fuel,T_average) -> Display8/1, Temperature Reactivity Feedback2/1(In1)
  [TH2] -> Reactor Thermal-Hydraulics Zone 3/3(T_c)
  Reactor Thermal-Hydraulics Zone 3/2(T_hot) -> T_hot/1, [TH3]
  Temperature Reactivity Feedback2/1(Out1) -> Sum2/2
  Demux2/1 -> Delay4/1
  Sum2/1 -> Zone 3 Kinetics1/6(rho_temp), Display1/1
  [mdot] -> Reactor Thermal-Hydraulics Zone 3/2(m_dot -mass flow in)
  Delay5/1 -> [dn1]
  Demux2/2 -> Delay2/1
  Reactor Thermal-Hydraulics Zone 2/2(T_hot) -> [TH2]
  Demux10/1 -> Delay/1
  Demux10/2 -> Delay3/1
  Delay4/1 -> [pn3]
  Delay/1 -> [pn2]
  Delay1/1 -> [pn1]
  Delay3/1 -> [dn2]
  Delay2/1 -> [dn3]
  [rodreactivityUpper] -> Sum2/1
  [pn1] -> Zone 2 Kinetics1/1(PROMPTN1)
  [pn3] -> Zone 2 Kinetics1/2(PROMPTN2)
  [dn3] -> Zone 2 Kinetics1/4(DELAYEDN2)
  [dn1] -> Zone 2 Kinetics1/3(DELAYEDN1)
  [pn2] -> Zone 1 Kinetics1/1(PROMPTN1)
  [pn3] -> Zone 1 Kinetics1/2(PROMPTN2)
  [dn2] -> Zone 1 Kinetics1/3(DELAYEDN1)
  [dn3] -> Zone 1 Kinetics1/4(DELAYEDN2)
  [pn3] -> Reactor Thermal-Hydraulics Zone 3/1(Q_rx)
  [pn2] -> Reactor Thermal-Hydraulics Zone 2/1(Q_rx)
  [pn1] -> Reactor Thermal-Hydraulics Zone 1/1(Q_rx)
  Mux1/1 -> Zonal Normalized Power/1, Normalized Power in Each Zone/1
  [pn1] -> Mux1/3  "Neutron 1"
  [pn3] -> Mux1/1  "Neutron 3"
  [pn2] -> Mux1/2  "Neutron 2"
  [TH1] -> Mux/3  "Tout RX1"
  [TH2] -> Mux/2  "Tout RX2"
  [TH3] -> Mux/1  "Tout RX3"
  Constant4/1 -> Product/1
  [mdot] -> Product/2
  Sum3/1 -> Product/3
  [TH3] -> Sum3/1
  [Tin] -> Reactor Thermal-Hydraulics Zone 1/3(T_c)
  [Tin] -> Sum3/2
  Product/1 -> W to MW/1
  W to MW/1 -> Thermal Power Extraction/1, Thermal Power Extracted/1
  [pn1] -> Sum4/1  "Neutron 1"
  [pn3] -> Sum4/3  "Neutron 3"
  [pn2] -> Sum4/2  "Neutron 2"
  Sum4/1 -> Gain1/1
  Gain1/1 -> Normalized Power Out of Reactor/1, Normalized Total Core Power/1
  Constant6/1 -> MATLAB Function/4(breaks)
  Constant3/1 -> MATLAB Function/3(DarkUpperCoeffs)
  Constant1/1 -> MATLAB Function/2(DarkMiddleCoeffs)
  Constant/1 -> MATLAB Function/1(DarkLowerCoeffs)
  MATLAB Function/1(RodWorthLower) -> Saturation/1
  MATLAB Function/2(RodWorthMiddle) -> Saturation1/1
  MATLAB Function/3(RodWorthUpper) -> Saturation2/1
  % Rod Withdrawn/1 -> MATLAB Function/5(RodWithdrawn)
  Saturation/1 -> Mux2/1, Dark Rod Worth FullyInserted 1/1, Display9/1
  Saturation1/1 -> Dark Rod Worth FullyInserted 2/1, Mux3/1, Display10/1
  Saturation2/1 -> Mux4/1, Dark Rod Worth FullyInserted 3/1, Display11/1
  Dark Rod Worth FullyInserted 1/1 -> Mux2/2, [rodreactivityLower]
  Dark Rod Worth FullyInserted 2/1 -> Mux3/2, [rodreactivityMiddle]
  Dark Rod Worth FullyInserted 3/1 -> Mux4/2, [rodreactivityUpper]
  Primary Mass Flowrate/1 -> [mdot]
  Primary Coolant Temperature In/1 -> [Tin]
  Mux2/1 -> Lower Zone Rod Worth and Reactivity/1
  Mux3/1 -> Middle Zone Rod Worth and Reactivity/1
  Mux4/1 -> Upper Zone Rod Worth and Reactivity/1
  Integrator4/1 -> Zone 3 Kinetics1/7(x)
  Zone 3 Kinetics1/2(xdot) -> Integrator4/1
  [pkeparams] -> Zone 3 Kinetics1/5(pkeparams)
  [dn2] -> Zone 3 Kinetics1/4(DELAYEDN2)
  [dn1] -> Zone 3 Kinetics1/3(DELAYEDN1)
  [pn2] -> Zone 3 Kinetics1/2(PROMPTN2)
  [pn1] -> Zone 3 Kinetics1/1(PROMPTN1)
  Zone 3 Kinetics1/1(y) -> Demux2/1
  Zone 2 Kinetics1/2(xdot) -> Integrator1/1
  Integrator1/1 -> Zone 2 Kinetics1/7(x)
  Zone 2 Kinetics1/1(y) -> Demux10/1
  Zone 1 Kinetics1/2(xdot) -> Integrator2/1
  Integrator2/1 -> Zone 1 Kinetics1/7(x)

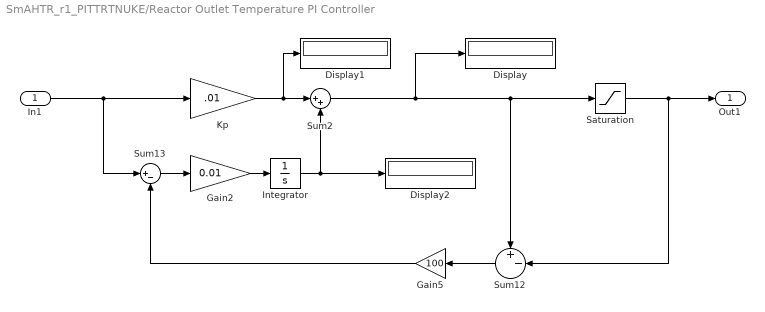
== system SmAHTR_r1_PITTRTNUKE/Reactor Outlet Temperature PI Controller ==
  In1 : Inport
  Display : Display
  Display1 : Display
  Display2 : Display
  Gain2 : Gain  Gain=0.01
  Gain5 : Gain  Gain=100
  Integrator : Integrator
  Kp : Gain  Gain=.01
  Saturation : Saturate  UpperLimit=1  LowerLimit=0
  Sum12 : Sum  Inputs=+-|
  Sum13 : Sum  Inputs=|+-
  Sum2 : Sum  Inputs=|++
  Out1 : Outport
  wires:
  In1/1 -> Kp/1, Sum13/1
  Sum2/1 -> Display/1, Sum12/1, Saturation/1
  Gain2/1 -> Integrator/1
  Integrator/1 -> Display2/1, Sum2/2
  Kp/1 -> Display1/1, Sum2/1
  Saturation/1 -> Sum12/2, Out1/1
  Sum12/1 -> Gain5/1
  Sum13/1 -> Gain2/1
  Gain5/1 -> Sum13/2

== system SmAHTR_r1_PITTRTNUKE/Salt Vault ==
  SHX Mass Flow : Inport
  Brayton Mass Flow : Inport  Port=2
  SHX Inlet Temperature : Inport  Port=3
  Brayton Inlet Temperature : Inport  Port=4
  Ambient Temperatre : Inport  Port=5
  Demux : Demux  Outputs=3
  From Workspace : FromWorkspace  VariableName=[0,V_secondary,rho_secondary,cps,rhoCO2]  SampleTime=0
  Integrator1 : Integrator  InitialCondition=SaltVaultICs
  Salt Vault : MATLAB Function  TreatAsAtomicUnit=on
  T_SHX Return : Outport
  T_salt : Outport  Port=2
  T_to Brayton : Outport  Port=3
  wires:
  Integrator1/1 -> Salt Vault/7(x)
  Brayton Inlet Temperature/1 -> Salt Vault/4(T_t1)
  Salt Vault/2(x_dot) -> Integrator1/1
  SHX Inlet Temperature/1 -> Salt Vault/3(T_s1)
  SHX Mass Flow/1 -> Salt Vault/1(mdots)
  Brayton Mass Flow/1 -> Salt Vault/2(mdott)
  Demux/1 -> T_SHX Return/1  "T_SHX return"
  Demux/2 -> T_salt/1  "T_salt"
  Salt Vault/1(y) -> Demux/1
  Demux/3 -> T_to Brayton/1
  From Workspace/1 -> Salt Vault/5(constants)
  Ambient Temperatre/1 -> Salt Vault/6(Tamb)

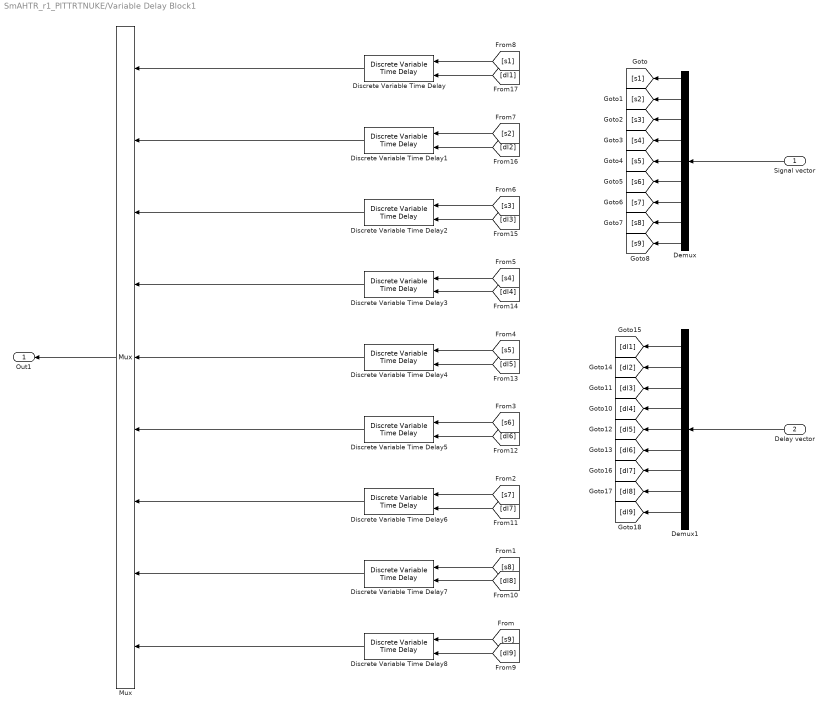
== system SmAHTR_r1_PITTRTNUKE/Variable Delay Block1 ==
  Signal vector : Inport
  Delay vector : Inport  Port=2
  Demux : Demux  Outputs=9
  Demux1 : Demux  Outputs=9
  Discrete Variable Time Delay{,1..8} (9 alike) : powerlib_meascontrol/Additional Components/Discrete Variable Time Delay  MaxDelay=1  InitialValue=0  Ts=delta_t  DFT=on
  Mux : Mux  Inputs=9
  Out1 : Outport
  wires:
  Discrete Variable Time Delay1/1 -> Mux/2
  Discrete Variable Time Delay/1 -> Mux/1
  Signal vector/1 -> Demux/1
  Delay vector/1 -> Demux1/1
  Discrete Variable Time Delay2/1 -> Mux/3
  Discrete Variable Time Delay3/1 -> Mux/4
  Discrete Variable Time Delay4/1 -> Mux/5
  Discrete Variable Time Delay5/1 -> Mux/6
  Discrete Variable Time Delay6/1 -> Mux/7
  Discrete Variable Time Delay7/1 -> Mux/8
  Discrete Variable Time Delay8/1 -> Mux/9
  Mux/1 -> Out1/1
  Demux/1 -> [s1]
  Demux/9 -> [s9]
  Demux/8 -> [s8]
  Demux/7 -> [s7]
  Demux/6 -> [s6]
  Demux/5 -> [s5]
  Demux/4 -> [s4]
  Demux/3 -> [s3]
  Demux/2 -> [s2]
  [s1] -> Discrete Variable Time Delay/1
  [s2] -> Discrete Variable Time Delay1/1
  [s3] -> Discrete Variable Time Delay2/1
  [s4] -> Discrete Variable Time Delay3/1
  [s5] -> Discrete Variable Time Delay4/1
  [s6] -> Discrete Variable Time Delay5/1
  [s7] -> Discrete Variable Time Delay6/1
  [s8] -> Discrete Variable Time Delay7/1
  [s9] -> Discrete Variable Time Delay8/1
  Demux1/9 -> [dl9]
  Demux1/1 -> [dl1]
  Demux1/2 -> [dl2]
  Demux1/3 -> [dl3]
  Demux1/4 -> [dl4]
  Demux1/5 -> [dl5]
  Demux1/6 -> [dl6]
  Demux1/7 -> [dl7]
  Demux1/8 -> [dl8]
  [dl1] -> Discrete Variable Time Delay/2
  [dl2] -> Discrete Variable Time Delay1/2
  [dl3] -> Discrete Variable Time Delay2/2
  [dl4] -> Discrete Variable Time Delay3/2
  [dl5] -> Discrete Variable Time Delay4/2
  [dl6] -> Discrete Variable Time Delay5/2
  [dl7] -> Discrete Variable Time Delay6/2
  [dl8] -> Discrete Variable Time Delay7/2
  [dl9] -> Discrete Variable Time Delay8/2

== system SmAHTR_r1_PITTRTNUKE/Primary Heat Exchanger Lumped Model #1/Cold side subsystem #N4 ==
  Tw : Inport
  Cold leg temp in : Inport  Port=2
  Cold leg mass flow in : Inport  Port=3
  Integrator : Integrator  InitialCondition=Ts_i
  Kc1 : Gain  Gain=Kc1
  Kc2 : Gain  Gain=Kc2
  Product : Product
  Sum : Sum  Inputs=|+-
  Sum1 : Sum  Inputs=++|
  Sum2 : Sum  Inputs=|+-
  Cold leg temp out : Outport
  Cold leg mass flow out : Outport  Port=2
  wires:
  Cold leg temp in/1 -> Sum/1
  Integrator/1 -> Sum/2, Cold leg temp out/1, Sum2/2
  Sum2/1 -> Kc2/1
  Sum/1 -> Product/1
  Kc2/1 -> Sum1/1
  Sum1/1 -> Integrator/1
  Cold leg mass flow in/1 -> Cold leg mass flow out/1, Product/2
  Product/1 -> Kc1/1
  Kc1/1 -> Sum1/2
  Tw/1 -> Sum2/1

== system SmAHTR_r1_PITTRTNUKE/Primary Heat Exchanger Lumped Model #1/HX wall4 ==
  Hot leg temp in : Inport
  Cold leg temp in : Inport  Port=2
  Integrator : Integrator  InitialCondition=Tw_i
  Kw1 : Gain  Gain=Kw1
  Kw2 : Gain  Gain=Kw2
  Kw3 : Gain  Gain=Kw3
  Sum : Sum  Inputs=|+-
  Sum1 : Sum  Inputs=|+-
  Sum2 : Sum  Inputs=+-|
  Twout : Outport
  wires:
  Sum2/1 -> Kw2/1
  Hot leg temp in/1 -> Sum/1
  Sum1/1 -> Kw3/1
  Cold leg temp in/1 -> Sum2/2
  Sum/1 -> Kw1/1
  Kw1/1 -> Sum1/1
  Kw3/1 -> Integrator/1
  Integrator/1 -> Twout/1, Sum2/1, Sum/2
  Kw2/1 -> Sum1/2

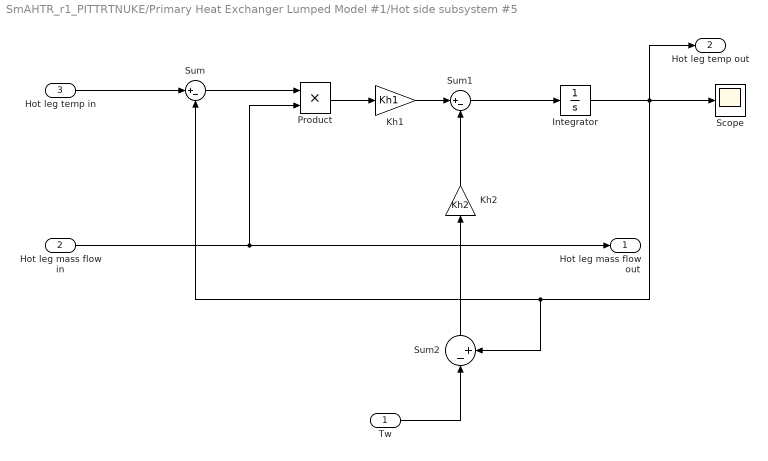
== system SmAHTR_r1_PITTRTNUKE/Primary Heat Exchanger Lumped Model #1/Hot side subsystem #5 ==
  Tw : Inport
  Hot leg mass flow in : Inport  Port=2
  Hot leg temp in : Inport  Port=3
  Integrator : Integrator  InitialCondition=Tp_i
  Kh1 : Gain  Gain=Kh1
  Kh2 : Gain  Gain=Kh2
  Product : Product
  Scope : Scope
  Sum : Sum  Inputs=|+-
  Sum1 : Sum  Inputs=|+-
  Sum2 : Sum  Inputs=|-+
  Hot leg mass flow out : Outport
  Hot leg temp out : Outport  Port=2
  wires:
  Product/1 -> Kh1/1
  Kh1/1 -> Sum1/1
  Sum1/1 -> Integrator/1
  Sum2/1 -> Kh2/1
  Kh2/1 -> Sum1/2
  Tw/1 -> Sum2/1
  Hot leg temp in/1 -> Sum/1
  Hot leg mass flow in/1 -> Hot leg mass flow out/1, Product/2
  Sum/1 -> Product/1
  Integrator/1 -> Hot leg temp out/1, Scope/1, Sum2/2, Sum/2

== system SmAHTR_r1_PITTRTNUKE/Primary Heat Exchanger Lumped Model #1/Secondary-side RCP Dynamics #1 ==
  In1 : Inport
  Digital Clock #1 : DigitalClock  SampleTime=.001
  RCP #1 : TransferFcn  Numerator=[rcpt]  Denominator=[1 rcpt]
  RCP Dynamics Switch #1 : Switch  Threshold=rcp_activatetime
  Out1 : Outport
  wires:
  In1/1 -> RCP #1/1, RCP Dynamics Switch #1/3
  Digital Clock #1/1 -> RCP Dynamics Switch #1/2
  RCP #1/1 -> RCP Dynamics Switch #1/1
  RCP Dynamics Switch #1/1 -> Out1/1

== system SmAHTR_r1_PITTRTNUKE/Primary Heat Exchanger Lumped Model #2/Cold side subsystem #N4 ==
  Tw : Inport
  Cold leg temp in : Inport  Port=2
  Cold leg mass flow in : Inport  Port=3
  Integrator : Integrator  InitialCondition=Ts_i
  Kc1 : Gain  Gain=Kc1
  Kc2 : Gain  Gain=Kc2
  Product : Product
  Sum : Sum  Inputs=|+-
  Sum1 : Sum  Inputs=++|
  Sum2 : Sum  Inputs=|+-
  Cold leg temp out : Outport
  Cold leg mass flow out : Outport  Port=2
  wires:
  Cold leg temp in/1 -> Sum/1
  Integrator/1 -> Sum/2, Cold leg temp out/1, Sum2/2
  Sum2/1 -> Kc2/1
  Sum/1 -> Product/1
  Kc2/1 -> Sum1/1
  Sum1/1 -> Integrator/1
  Cold leg mass flow in/1 -> Cold leg mass flow out/1, Product/2
  Product/1 -> Kc1/1
  Kc1/1 -> Sum1/2
  Tw/1 -> Sum2/1

== system SmAHTR_r1_PITTRTNUKE/Primary Heat Exchanger Lumped Model #2/HX wall4 ==
  Hot leg temp in : Inport
  Cold leg temp in : Inport  Port=2
  Integrator : Integrator  InitialCondition=Tw_i
  Kw1 : Gain  Gain=Kw1
  Kw2 : Gain  Gain=Kw2
  Kw3 : Gain  Gain=Kw3
  Sum : Sum  Inputs=|+-
  Sum1 : Sum  Inputs=|+-
  Sum2 : Sum  Inputs=+-|
  Twout : Outport
  wires:
  Sum2/1 -> Kw2/1
  Hot leg temp in/1 -> Sum/1
  Sum1/1 -> Kw3/1
  Cold leg temp in/1 -> Sum2/2
  Sum/1 -> Kw1/1
  Kw1/1 -> Sum1/1
  Kw3/1 -> Integrator/1
  Integrator/1 -> Twout/1, Sum2/1, Sum/2
  Kw2/1 -> Sum1/2

== system SmAHTR_r1_PITTRTNUKE/Primary Heat Exchanger Lumped Model #2/Hot side subsystem #5 ==
  Tw : Inport
  Hot leg mass flow in : Inport  Port=2
  Hot leg temp in : Inport  Port=3
  Integrator : Integrator  InitialCondition=Tp_i
  Kh1 : Gain  Gain=Kh1
  Kh2 : Gain  Gain=Kh2
  Product : Product
  Scope : Scope
  Sum : Sum  Inputs=|+-
  Sum1 : Sum  Inputs=|+-
  Sum2 : Sum  Inputs=|-+
  Hot leg mass flow out : Outport
  Hot leg temp out : Outport  Port=2
  wires:
  Product/1 -> Kh1/1
  Kh1/1 -> Sum1/1
  Sum1/1 -> Integrator/1
  Sum2/1 -> Kh2/1
  Kh2/1 -> Sum1/2
  Tw/1 -> Sum2/1
  Hot leg temp in/1 -> Sum/1
  Hot leg mass flow in/1 -> Hot leg mass flow out/1, Product/2
  Sum/1 -> Product/1
  Integrator/1 -> Hot leg temp out/1, Scope/1, Sum2/2, Sum/2

== system SmAHTR_r1_PITTRTNUKE/Primary Heat Exchanger Lumped Model #2/Secondary-side RCP Dynamics #2 ==
  In1 : Inport
  Digital Clock#2 : DigitalClock  SampleTime=.001
  RCP #2 : TransferFcn  Numerator=[rcpt]  Denominator=[1 rcpt]
  RCP Dynamics Switch #2 : Switch  Threshold=rcp_activatetime
  Out1 : Outport
  wires:
  RCP Dynamics Switch #2/1 -> Out1/1
  In1/1 -> RCP #2/1, RCP Dynamics Switch #2/3
  Digital Clock#2/1 -> RCP Dynamics Switch #2/2
  RCP #2/1 -> RCP Dynamics Switch #2/1

== system SmAHTR_r1_PITTRTNUKE/Primary Heat Exchanger Lumped Model #3/Cold side subsystem #N4 ==
  Tw : Inport
  Cold leg temp in : Inport  Port=2
  Cold leg mass flow in : Inport  Port=3
  Integrator : Integrator  InitialCondition=Ts_i
  Kc1 : Gain  Gain=Kc1
  Kc2 : Gain  Gain=Kc2
  Product : Product
  Sum : Sum  Inputs=|+-
  Sum1 : Sum  Inputs=++|
  Sum2 : Sum  Inputs=|+-
  Cold leg temp out : Outport
  Cold leg mass flow out : Outport  Port=2
  wires:
  Cold leg temp in/1 -> Sum/1
  Integrator/1 -> Sum/2, Cold leg temp out/1, Sum2/2
  Sum2/1 -> Kc2/1
  Sum/1 -> Product/1
  Kc2/1 -> Sum1/1
  Sum1/1 -> Integrator/1
  Cold leg mass flow in/1 -> Cold leg mass flow out/1, Product/2
  Product/1 -> Kc1/1
  Kc1/1 -> Sum1/2
  Tw/1 -> Sum2/1

== system SmAHTR_r1_PITTRTNUKE/Primary Heat Exchanger Lumped Model #3/HX wall4 ==
  Hot leg temp in : Inport
  Cold leg temp in : Inport  Port=2
  Integrator : Integrator  InitialCondition=Tw_i
  Kw1 : Gain  Gain=Kw1
  Kw2 : Gain  Gain=Kw2
  Kw3 : Gain  Gain=Kw3
  Sum : Sum  Inputs=|+-
  Sum1 : Sum  Inputs=|+-
  Sum2 : Sum  Inputs=+-|
  Twout : Outport
  wires:
  Sum2/1 -> Kw2/1
  Hot leg temp in/1 -> Sum/1
  Sum1/1 -> Kw3/1
  Cold leg temp in/1 -> Sum2/2
  Sum/1 -> Kw1/1
  Kw1/1 -> Sum1/1
  Kw3/1 -> Integrator/1
  Integrator/1 -> Twout/1, Sum2/1, Sum/2
  Kw2/1 -> Sum1/2

== system SmAHTR_r1_PITTRTNUKE/Primary Heat Exchanger Lumped Model #3/Hot side subsystem #5 ==
  Tw : Inport
  Hot leg mass flow in : Inport  Port=2
  Hot leg temp in : Inport  Port=3
  Integrator : Integrator  InitialCondition=Tp_i
  Kh1 : Gain  Gain=Kh1
  Kh2 : Gain  Gain=Kh2
  Product : Product
  Scope : Scope
  Sum : Sum  Inputs=|+-
  Sum1 : Sum  Inputs=|+-
  Sum2 : Sum  Inputs=|-+
  Hot leg mass flow out : Outport
  Hot leg temp out : Outport  Port=2
  wires:
  Product/1 -> Kh1/1
  Kh1/1 -> Sum1/1
  Sum1/1 -> Integrator/1
  Sum2/1 -> Kh2/1
  Kh2/1 -> Sum1/2
  Tw/1 -> Sum2/1
  Hot leg temp in/1 -> Sum/1
  Hot leg mass flow in/1 -> Hot leg mass flow out/1, Product/2
  Sum/1 -> Product/1
  Integrator/1 -> Hot leg temp out/1, Scope/1, Sum2/2, Sum/2

== system SmAHTR_r1_PITTRTNUKE/Primary Heat Exchanger Lumped Model #3/Secondary-side RCP Dynamics #3 ==
  In1 : Inport
  Digital Clock #3 : DigitalClock  SampleTime=.001
  RCP #3 : TransferFcn  Numerator=[rcpt]  Denominator=[1 rcpt]
  RCP Dynamics Switch #3 : Switch  Threshold=rcp_activatetime
  Out1 : Outport
  wires:
  RCP #3/1 -> RCP Dynamics Switch #3/1
  Digital Clock #3/1 -> RCP Dynamics Switch #3/2
  In1/1 -> RCP #3/1, RCP Dynamics Switch #3/3
  RCP Dynamics Switch #3/1 -> Out1/1

== system SmAHTR_r1_PITTRTNUKE/Reactor Kinetics and Thermal Hydraulics/Reactor Thermal-Hydraulics Zone 1 ==
  Q_rx : Inport
  m_dot -mass flow in : Inport  Port=2
  T_c : Inport  Port=3
  Demux : Demux  Outputs=3
  From Workspace : FromWorkspace  VariableName=[0,cpc,cpf,mc,mf,uh,Ar]  SampleTime=0
  Integrator1 : Integrator  InitialCondition=[1047;658.6]
  MATLAB Function : MATLAB Function  TreatAsAtomicUnit=on
  Mux : Mux  Inputs=2
  Scope : Scope
      settings: SaveName=ScopeData8
  Scope1 : Scope
      settings: SaveName=ScopeData9
  Scope2 : Scope
      settings: SaveName=ScopeData2
  T_fuel,T_average : Outport
  T_hot : Outport  Port=2
  wires:
  MATLAB Function/2(x_dot) -> Integrator1/1
  Integrator1/1 -> MATLAB Function/5(x)
  m_dot -mass flow in/1 -> MATLAB Function/1(m_dot)
  Demux/2 -> Scope1/1, Mux/2  "T_average"
  T_c/1 -> MATLAB Function/4(T_c)
  From Workspace/1 -> MATLAB Function/3(constants)
  Q_rx/1 -> MATLAB Function/2(Q_rx)
  MATLAB Function/1(y) -> Demux/1
  Demux/1 -> Mux/1  "T_fuel"
  Mux/1 -> Scope2/1, T_fuel,T_average/1
  Demux/3 -> T_hot/1, Scope/1  "T_hot"

== system SmAHTR_r1_PITTRTNUKE/Reactor Kinetics and Thermal Hydraulics/Reactor Thermal-Hydraulics Zone 2 ==
  Q_rx : Inport
  m_dot -mass flow in : Inport  Port=2
  T_c : Inport  Port=3
  Demux : Demux  Outputs=3
  From Workspace : FromWorkspace  VariableName=[0,cpc,cpf,mc,mf,uh,Ar]  SampleTime=0
  Integrator1 : Integrator  InitialCondition=[1101;676.6]
  MATLAB Function : MATLAB Function  TreatAsAtomicUnit=on
  Mux : Mux  Inputs=2
  Scope : Scope
      settings: SaveName=ScopeData8
  Scope1 : Scope
      settings: SaveName=ScopeData9
  Scope2 : Scope
      settings: SaveName=ScopeData2
  T_fuel,T_average : Outport
  T_hot : Outport  Port=2
  wires:
  MATLAB Function/2(x_dot) -> Integrator1/1
  Integrator1/1 -> MATLAB Function/5(x)
  m_dot -mass flow in/1 -> MATLAB Function/1(m_dot)
  Demux/2 -> Scope1/1, Mux/2  "T_average"
  T_c/1 -> MATLAB Function/4(T_c)
  From Workspace/1 -> MATLAB Function/3(constants)
  Q_rx/1 -> MATLAB Function/2(Q_rx)
  MATLAB Function/1(y) -> Demux/1
  Demux/1 -> Mux/1  "T_fuel"
  Mux/1 -> Scope2/1, T_fuel,T_average/1
  Demux/3 -> T_hot/1, Scope/1  "T_hot"

== system SmAHTR_r1_PITTRTNUKE/Reactor Kinetics and Thermal Hydraulics/Reactor Thermal-Hydraulics Zone 3 ==
  Q_rx : Inport
  m_dot -mass flow in : Inport  Port=2
  T_c : Inport  Port=3
  Demux : Demux  Outputs=3
  From Workspace : FromWorkspace  VariableName=[0,cpc,cpf,mc,mf,uh,Ar]  SampleTime=0
  Integrator1 : Integrator  InitialCondition=[1061; 694.1]
  MATLAB Function : MATLAB Function  TreatAsAtomicUnit=on
  Mux : Mux  Inputs=2
  Scope : Scope
      settings: SaveName=ScopeData8
  Scope1 : Scope
      settings: SaveName=ScopeData9
  Scope2 : Scope
      settings: SaveName=ScopeData2
  T_fuel,T_average : Outport
  T_hot : Outport  Port=2
  wires:
  MATLAB Function/2(x_dot) -> Integrator1/1
  Integrator1/1 -> MATLAB Function/5(x)
  m_dot -mass flow in/1 -> MATLAB Function/1(m_dot)
  Demux/2 -> Scope1/1, Mux/2  "T_average"
  T_c/1 -> MATLAB Function/4(T_c)
  From Workspace/1 -> MATLAB Function/3(constants)
  Q_rx/1 -> MATLAB Function/2(Q_rx)
  MATLAB Function/1(y) -> Demux/1
  Demux/1 -> Mux/1  "T_fuel"
  Mux/1 -> Scope2/1, T_fuel,T_average/1
  Demux/3 -> T_hot/1, Scope/1  "T_hot"

== system SmAHTR_r1_PITTRTNUKE/Reactor Kinetics and Thermal Hydraulics/Temperature Reactivity Feedback1 ==
  In1 : Inport
  Sum : Sum  Inputs=|+-
  reactivity feedback matrix : Gain  Gain=alpha  Multiplication=Matrix(K*u)
  reactivity reference temperature : Constant  Value=xfc0  VectorParams1D=off
  Out1 : Outport
  wires:
  reactivity reference temperature/1 -> Sum/2
  Sum/1 -> reactivity feedback matrix/1
  reactivity feedback matrix/1 -> Out1/1
  In1/1 -> Sum/1

== system SmAHTR_r1_PITTRTNUKE/Reactor Kinetics and Thermal Hydraulics/Temperature Reactivity Feedback2 ==
  In1 : Inport
  Sum : Sum  Inputs=|+-
  reactivity feedback matrix : Gain  Gain=alpha  Multiplication=Matrix(K*u)
  reactivity reference temperature : Constant  Value=xfc0  VectorParams1D=off
  Out1 : Outport
  wires:
  reactivity reference temperature/1 -> Sum/2
  Sum/1 -> reactivity feedback matrix/1
  reactivity feedback matrix/1 -> Out1/1
  In1/1 -> Sum/1

== system SmAHTR_r1_PITTRTNUKE/Reactor Kinetics and Thermal Hydraulics/Temperature Reactivity Feedback3 ==
  In1 : Inport
  Sum : Sum  Inputs=|+-
  reactivity feedback matrix : Gain  Gain=alpha  Multiplication=Matrix(K*u)
  reactivity reference temperature : Constant  Value=xfc0  VectorParams1D=off
  Out1 : Outport
  wires:
  reactivity reference temperature/1 -> Sum/2
  Sum/1 -> reactivity feedback matrix/1
  reactivity feedback matrix/1 -> Out1/1
  In1/1 -> Sum/1
